simulink model "sampleModel1879"  (R2023a)
settings: Solver=VariableStepAuto  StartTime=0.0  StopTime=10.0  RelTol=1e-3
libraries: hdlsllib x4, simulink x1
settings Model: Creator=user1  LastModifiedBy=user1

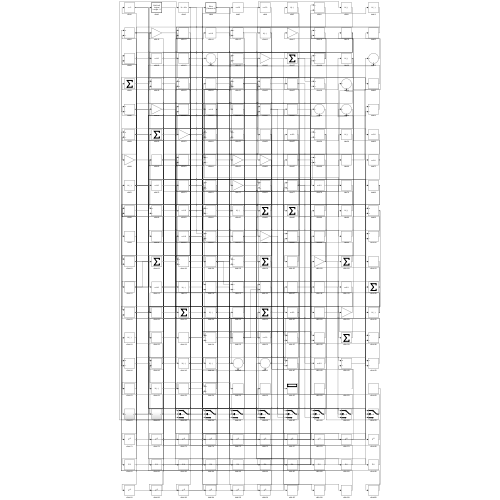
[thumbnail: Simulink's stored preview of the top-level diagram]
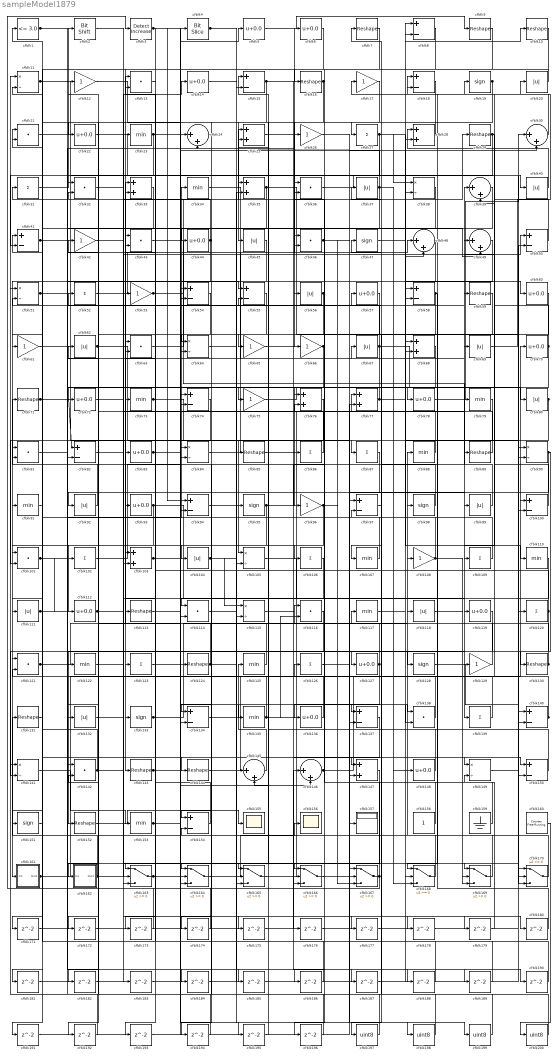
== system sampleModel1879 ==
  cfblk1 : hdlsllib/Logic and Bit Operations/Compare To Constant  relop=<=  const=3.0  OutDataTypeStr=boolean
  cfblk{7,9..10,16,29,59,71,85,89,113,124,130..131,143..144,152} (16 alike) : Reshape
  cfblk{8,15,18,41,50,54..55,58,74,82,94,97,100,134,137,140,150,154} (18 alike) : Sum  Inputs=+-
  cfblk{13,21,32,36,43,46,63,81,101,114,116,121,138,142} (14 alike) : DotProduct  OutDataTypeStr=Inherit: Inherit via internal rule
  cfblk{27,31,52,86..87,102,106,109,120,123,126,139} (12 alike) : Sum  Inputs=+
  cfblk{25,28,33,35,68,76..77,103,147} (9 alike) : Sum
  cfblk{20,37,40,45,56,62,67,69,80,92,99,104,111,118,132} (15 alike) : Abs  SaturateOnIntegerOverflow=off
  cfblk{11,38,51,64,84,90,105,115,141,149} (10 alike) : Product  Inputs=*/  RndMeth=Zero  SaturateOnIntegerOverflow=on
  cfblk{23,34,73,79,88,91,107,110,117,122,125,135,153} (13 alike) : MinMax
  cfblk{12,17,26,42,53,61,65..66,75,96,108,129} (12 alike) : Gain
  cfblk{5..6,14,22,44,57,60,70,72,78,83,93,112,119,127,136,148} (17 alike) : Bias  Bias=0.0  SaturateOnIntegerOverflow=off
  cfblk{19,47,95,98,128,133,151} (7 alike) : Signum
  cfblk{24,30,39,48..49,145..146} (7 alike) : Sum  Inputs=|++
  cfblk155 : Scope
  cfblk156 : Scope
  cfblk157 : Display
  cfblk158 : Constant  SampleTime=-1
  cfblk159 : Ground
  cfblk160 : hdlsllib/Sources/Counter Free-Running  NumBits=16  tsamp=-1
  cfblk161 : Subsystem
      settings: LibrarySourceBlock=|
      | hdlsllib/Ports &
      | Subsystems/Subsystem
  cfblk162 : Subsystem
      settings: LibrarySourceBlock=|
      | hdlsllib/Ports &
      | Subsystems/Subsystem
  cfblk{163..170} (8 alike) : Switch  SaturateOnIntegerOverflow=off  InputSameDT=off
  cfblk{171..196} (26 alike) : Delay  SampleTime=1
  cfblk{197..200} (4 alike) : DataTypeConversion  OutDataTypeStr=uint8  SaturateOnIntegerOverflow=off  RndMeth=Floor
  cfblk2 : hdlsllib/Logic and Bit Operations/Bit Shift  mode=Shift Left Logical  N=0
  cfblk3 : simulink/Logic and Bit Operations/Detect Increase  vinit=0.0  OutDataTypeStr=boolean
      settings: LibrarySourceBlock=|
      | hdlsllib/Logic and Bit
      | Operations/Detect
      | Increase
  cfblk4 : hdlsllib/Logic and Bit Operations/Bit Slice  lidx=7  ridx=0
  wires:
  cfblk19/1 -> cfblk66/1, cfblk145/2, cfblk101/1
  cfblk104/1 -> cfblk115/1, cfblk79/1, cfblk169/3
  cfblk74/1 -> cfblk161/1(In1)
  cfblk165/1 -> cfblk77/1
  cfblk34/1 -> cfblk67/1
  cfblk145/1 -> cfblk125/1
  cfblk61/1 -> cfblk96/1
  cfblk130/1 -> cfblk70/1, cfblk36/1
  cfblk43/1 -> cfblk139/1
  cfblk76/1 -> cfblk105/1
  cfblk54/1 -> cfblk143/1
  cfblk163/1 -> cfblk59/1, cfblk13/2, cfblk177/1
  cfblk75/1 -> cfblk78/1
  cfblk96/1 -> cfblk112/1, cfblk167/3
  cfblk5/1 -> cfblk9/1
  cfblk48/1 -> cfblk91/1
  cfblk93/1 -> cfblk121/1, cfblk167/1, cfblk76/2
  cfblk10/1 -> cfblk86/1
  cfblk56/1 -> cfblk132/1, cfblk64/1, cfblk174/1
  cfblk7/1 -> cfblk133/1
  cfblk162/1(Out1) -> cfblk131/1, cfblk69/1
  cfblk124/1 -> cfblk33/1, cfblk170/2
  cfblk139/1 -> cfblk88/1
  cfblk121/1 -> cfblk127/1, cfblk24/1
  cfblk167/1 -> cfblk3/1, cfblk74/2
  cfblk91/1 -> cfblk151/1
  cfblk8/1 -> cfblk111/1
  cfblk161/1(Out1) -> cfblk126/1, cfblk94/2
  cfblk40/1 -> cfblk28/1
  cfblk109/1 -> cfblk34/1
  cfblk69/1 -> cfblk20/1
  cfblk11/1 -> cfblk83/1, cfblk44/1
  cfblk17/1 -> cfblk154/1
  cfblk59/1 -> cfblk107/1
  cfblk27/1 -> cfblk38/1, cfblk41/2, cfblk114/2, cfblk110/1
  cfblk16/1 -> cfblk45/1, cfblk193/1
  cfblk168/1 -> cfblk98/1
  cfblk44/1 -> cfblk113/1, cfblk103/2, cfblk21/1
  cfblk142/1 -> cfblk50/1, cfblk41/1
  cfblk13/1 -> cfblk123/1
  cfblk31/1 -> cfblk2/1
  cfblk84/1 -> cfblk6/1
  cfblk102/1 -> cfblk4/1
  cfblk129/1 -> cfblk108/1
  cfblk144/1 -> cfblk100/1
  cfblk71/1 -> cfblk82/1, cfblk64/2, cfblk128/1, cfblk166/3
  cfblk62/1 -> cfblk157/1, cfblk166/2
  cfblk55/1 -> cfblk65/1
  cfblk90/1 -> cfblk130/1, cfblk163/3
  cfblk92/1 -> cfblk71/1
  cfblk1/1 -> cfblk55/1, cfblk166/1
  cfblk151/1 -> cfblk11/2
  cfblk22/1 -> cfblk85/1
  cfblk134/1 -> cfblk58/1
  cfblk107/1 -> cfblk63/1
  cfblk110/1 -> cfblk114/1
  cfblk105/1 -> cfblk119/1
  cfblk65/1 -> cfblk149/1
  cfblk20/1 -> cfblk16/1
  cfblk99/1 -> cfblk39/1
  cfblk63/1 -> cfblk25/1
  cfblk35/1 -> cfblk100/2, cfblk104/1, cfblk147/1
  cfblk86/1 -> cfblk15/1
  cfblk53/1 -> cfblk29/1, cfblk165/3
  cfblk60/1 -> cfblk76/1
  cfblk111/1 -> cfblk48/1, cfblk46/1, cfblk102/1
  cfblk146/1 -> cfblk68/1, cfblk116/1
  cfblk103/1 -> cfblk33/2, cfblk185/1
  cfblk118/1 -> cfblk150/1
  cfblk36/1 -> cfblk40/1
  cfblk89/1 -> cfblk47/1
  cfblk95/1 -> cfblk89/1, cfblk122/1
  cfblk135/1 -> cfblk137/1, cfblk116/2, cfblk21/2
  cfblk170/1 -> cfblk84/1
  cfblk78/1 -> cfblk30/1
  cfblk26/1 -> cfblk137/2
  cfblk77/1 -> cfblk90/2, cfblk72/1, cfblk148/1
  cfblk152/1 -> cfblk155/1
  cfblk112/1 -> cfblk14/1, cfblk188/1
  cfblk138/1 -> cfblk12/1
  cfblk100/1 -> cfblk19/1
  cfblk9/1 -> cfblk15/2
  cfblk125/1 -> cfblk42/1
  cfblk21/1 -> cfblk140/1
  cfblk18/1 -> cfblk136/1
  cfblk149/1 -> cfblk120/1
  cfblk6/1 -> cfblk23/1
  cfblk119/1 -> cfblk152/1
  cfblk164/1 -> cfblk156/1
  cfblk169/1 -> cfblk62/1
  cfblk133/1 -> cfblk118/1, cfblk30/2
  cfblk88/1 -> cfblk52/1
  cfblk41/1 -> cfblk80/1, cfblk26/1
  cfblk29/1 -> cfblk165/1, cfblk109/1
  cfblk47/1 -> cfblk60/1
  cfblk154/1 -> cfblk93/1
  cfblk57/1 -> cfblk84/2
  cfblk66/1 -> cfblk163/1, cfblk164/3, cfblk182/1
  cfblk3/1 -> cfblk103/1, cfblk94/1, cfblk49/2
  cfblk32/1 -> cfblk115/2
  cfblk38/1 -> cfblk61/1
  cfblk73/1 -> cfblk95/1, cfblk169/1
  cfblk30/1 -> cfblk18/1
  cfblk128/1 -> cfblk170/1
  cfblk80/1 -> cfblk105/2, cfblk101/2
  cfblk68/1 -> cfblk87/1
  cfblk23/1 -> cfblk180/1, cfblk181/1
  cfblk67/1 -> cfblk150/2, cfblk31/1, cfblk106/1
  cfblk12/1 -> cfblk124/1
  cfblk79/1 -> cfblk82/2
  cfblk140/1 -> cfblk51/2, cfblk49/1
  cfblk37/1 -> cfblk144/1, cfblk168/3, cfblk24/2
  cfblk70/1 -> cfblk39/2, cfblk134/1
  cfblk33/1 -> cfblk92/1
  cfblk58/1 -> cfblk168/1, cfblk147/2
  cfblk82/1 -> cfblk74/1
  cfblk141/1 -> cfblk153/1
  cfblk117/1 -> cfblk10/1
  cfblk127/1 -> cfblk43/1, cfblk196/1
  cfblk143/1 -> cfblk5/1, cfblk169/2
  cfblk87/1 -> cfblk142/1
  cfblk83/1 -> cfblk135/1, cfblk36/2
  cfblk14/1 -> cfblk145/1
  cfblk52/1 -> cfblk8/1
  cfblk15/1 -> cfblk162/1(In1), cfblk190/1
  cfblk120/1 -> cfblk141/2, cfblk13/1
  cfblk101/1 -> cfblk46/2, cfblk184/1
  cfblk46/1 -> cfblk99/1, cfblk167/2
  cfblk24/1 -> cfblk164/1
  cfblk108/1 -> cfblk57/1, cfblk170/3, cfblk81/2
  cfblk153/1 -> cfblk146/2, cfblk63/2
  cfblk123/1 -> cfblk138/1
  cfblk158/1 -> cfblk81/1
  cfblk51/1 -> cfblk53/1, cfblk164/2
  cfblk28/1 -> cfblk22/1, cfblk27/1
  cfblk2/1 -> cfblk75/1
  cfblk136/1 -> cfblk73/1
  cfblk148/1 -> cfblk117/1
  cfblk25/1 -> cfblk56/1
  cfblk81/1 -> cfblk54/1
  cfblk50/1 -> cfblk17/1
  cfblk4/1 -> cfblk38/2, cfblk138/2
  cfblk122/1 -> cfblk35/1
  cfblk98/1 -> cfblk7/1
  cfblk147/1 -> cfblk163/2
  cfblk72/1 -> cfblk129/1
  cfblk159/1 -> cfblk37/1
  cfblk150/1 -> cfblk25/2
  cfblk137/1 -> cfblk171/1
  cfblk171/1 -> cfblk48/2
  cfblk116/1 -> cfblk172/1
  cfblk172/1 -> cfblk146/1
  cfblk39/1 -> cfblk173/1
  cfblk173/1 -> cfblk51/1
  cfblk174/1 -> cfblk121/2
  cfblk132/1 -> cfblk175/1
  cfblk175/1 -> cfblk168/2
  cfblk115/1 -> cfblk176/1
  cfblk176/1 -> cfblk58/2
  cfblk177/1 -> cfblk90/1
  cfblk126/1 -> cfblk178/1
  cfblk178/1 -> cfblk50/2
  cfblk94/1 -> cfblk179/1
  cfblk179/1 -> cfblk149/2
  cfblk180/1 -> cfblk18/2
  cfblk181/1 -> cfblk134/2
  cfblk182/1 -> cfblk35/2
  cfblk42/1 -> cfblk183/1
  cfblk183/1 -> cfblk8/2
  cfblk184/1 -> cfblk68/2
  cfblk185/1 -> cfblk140/2
  cfblk49/1 -> cfblk186/1
  cfblk186/1 -> cfblk165/2
  cfblk85/1 -> cfblk187/1
  cfblk187/1 -> cfblk28/2
  cfblk188/1 -> cfblk142/2
  cfblk114/1 -> cfblk189/1
  cfblk189/1 -> cfblk1/1
  cfblk190/1 -> cfblk43/2
  cfblk131/1 -> cfblk191/1
  cfblk191/1 -> cfblk54/2
  cfblk45/1 -> cfblk192/1
  cfblk192/1 -> cfblk141/1
  cfblk193/1 -> cfblk77/2
  cfblk106/1 -> cfblk194/1
  cfblk194/1 -> cfblk11/1
  cfblk113/1 -> cfblk195/1
  cfblk195/1 -> cfblk55/2
  cfblk196/1 -> cfblk154/2
  cfblk97/1 -> cfblk197/1
  cfblk197/1 -> cfblk32/1
  cfblk64/1 -> cfblk198/1
  cfblk198/1 -> cfblk97/1
  cfblk166/1 -> cfblk199/1
  cfblk199/1 -> cfblk97/2
  cfblk160/1 -> cfblk200/1
  cfblk200/1 -> cfblk32/2

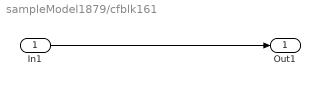
== system sampleModel1879/cfblk161 ==
  In1 : Inport
  Out1 : Outport
  wires:
  In1/1 -> Out1/1

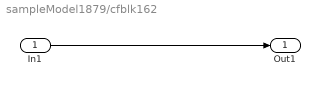
== system sampleModel1879/cfblk162 ==
  In1 : Inport
  Out1 : Outport
  wires:
  In1/1 -> Out1/1
